simulink model "FruitSorting_slice_vision"  (R2025a)
settings: Solver=FixedStepDiscrete  StartTime=0.0  StopTime=0.1  FixedStep=0.1  RelTol=1e-3
settings Model: Creator=Mugin  LastModifiedBy=Mugin

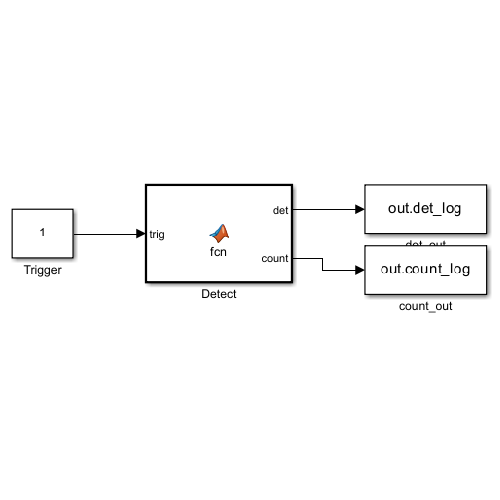
[thumbnail: Simulink's stored preview of the top-level diagram]
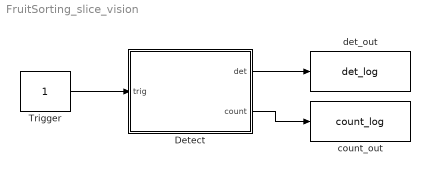
== system FruitSorting_slice_vision ==
  Detect : MATLAB Function  TreatAsAtomicUnit=on
  Trigger : Constant  SampleTime=0.1
  count_out : ToWorkspace  VariableName=count_log  SampleTime=-1
  det_out : ToWorkspace  VariableName=det_log  SampleTime=-1
  wires:
  Trigger/1 -> Detect/1(trig)
  Detect/1(det) -> det_out/1
  Detect/2(count) -> count_out/1

== matlab function FruitSorting_slice_vision/Detect ==
  data: trig input; det output; count output
function [det, count] = fcn(trig)
%#codegen
coder.extrinsic('py_detect_test');
det = zeros(8,5);
count = int32(0);
[det_tmp, cnt_tmp] = py_detect_test(trig);
det = double(det_tmp);
count = int32(cnt_tmp);
end
